simulink model "ControloPosicao2020b"  (R2022b)
settings: Solver=VariableStepAuto  StartTime=0.0  StopTime=10.0  RelTol=1e-3
libraries: fuzblock x12, slpidlib x4, dspswit3 x2
settings Model: Creator=jpmat  LastModifiedBy=jpmat
settings OptimizationCC: ReuseModelBlockBuffer=on

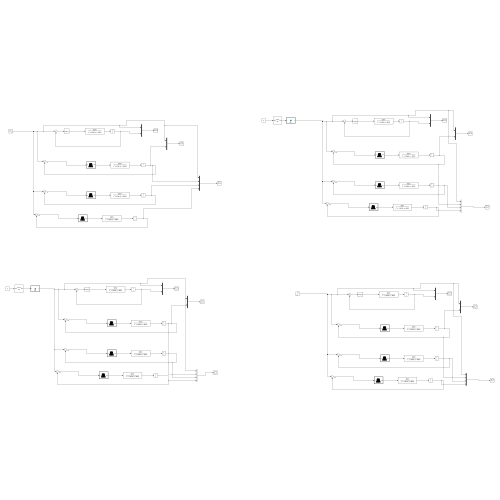
[thumbnail: Simulink's stored preview of the top-level diagram]
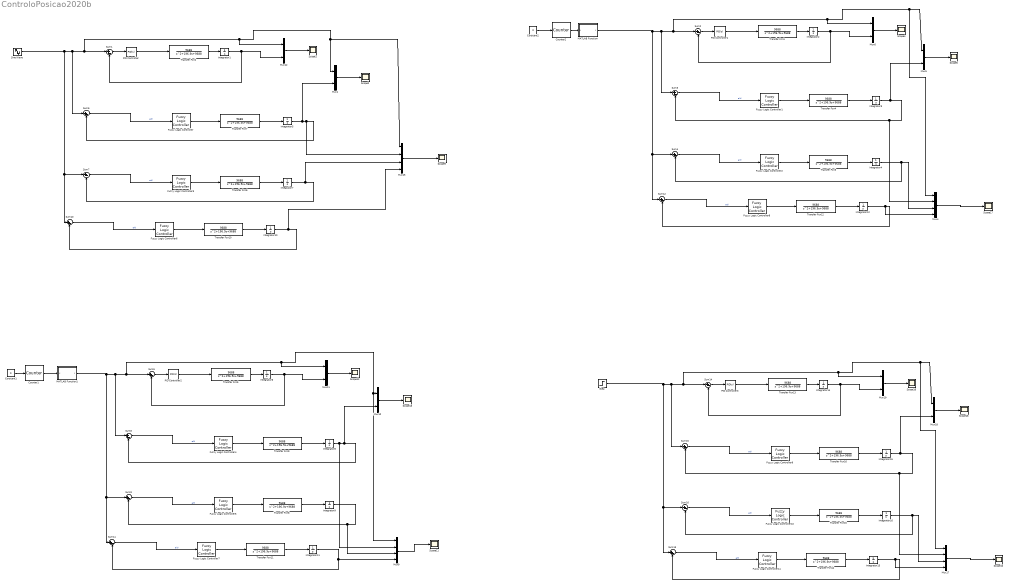
== system ControloPosicao2020b ==
  Constant1 : Constant  Value=0
  Constant2 : Constant  Value=0
  Counter1 : dspswit3/Counter  Direction=Up  CountEvent=Free running  CounterSize=User defined  MaxCount=10000000  InitialCount=0  Output=Count  HitValue=32  ResetInput=on  SamplesPerFrame=1  Ts=0.01  CntDtype=double  HitDtype=Logical
  Counter2 : dspswit3/Counter  Direction=Up  CountEvent=Free running  CounterSize=User defined  MaxCount=10000000  InitialCount=0  Output=Count  HitValue=32  ResetInput=on  SamplesPerFrame=1  Ts=0.01  CntDtype=double  HitDtype=Logical
  Fuzzy Logic Controller{,1,4,9} (4 alike) : fuzblock/Fuzzy Logic  Controller  FIS=posFIS  OutputSampleNumber=101  DataType=double  FuzzifiedInputs=off  RuleFiringStrengths=off  RuleOutputs=off  AggregatedOutputs=off  SimulateUsing=Interpreted execution  OutOfRangeInputValueMessage=warning  NoRuleFiredMessage=warning  EmptyOutputFuzzySetMessage=warning
  Fuzzy Logic Controller{2..3,5,10} (4 alike) : fuzblock/Fuzzy Logic  Controller  FIS=posFIS11  OutputSampleNumber=101  DataType=double  FuzzifiedInputs=off  RuleFiringStrengths=off  RuleOutputs=off  AggregatedOutputs=off  SimulateUsing=Interpreted execution  OutOfRangeInputValueMessage=warning  NoRuleFiredMessage=warning  EmptyOutputFuzzySetMessage=warning
  Fuzzy Logic Controller{6..8,11} (4 alike) : fuzblock/Fuzzy Logic  Controller  FIS=posFIS5  OutputSampleNumber=101  DataType=double  FuzzifiedInputs=off  RuleFiringStrengths=off  RuleOutputs=off  AggregatedOutputs=off  SimulateUsing=Interpreted execution  OutOfRangeInputValueMessage=warning  NoRuleFiredMessage=warning  EmptyOutputFuzzySetMessage=warning
  Integrator{1..16} (16 alike) : Integrator
  MATLAB Function : MATLAB Function  TreatAsAtomicUnit=on
  MATLAB Function1 : MATLAB Function  TreatAsAtomicUnit=on
  Mux{1,5..6,10..12,18..19} (8 alike) : Mux  Inputs=2
  Mux{4,9,15,17} (4 alike) : Mux
  PID Controller{,1..3} (4 alike) : slpidlib/PID Controller  Controller=PID  Form=Parallel  TimeDomain=Continuous-time  UseExternalTs=off  SampleTime=-1  IntegratorMethod=Forward Euler  FilterMethod=Forward Euler  ControllerParametersSource=internal  P=15  I=2  UseKiTs=off  D=0.05  N=100  UseFilter=on  TunerSelectOption=Transfer Function Based (PID Tuner App)  InitialConditionSource=internal  InitialConditionForIntegrator=0  InitialConditionForFilter=0  DifferentiatorICPrevScaledInput=0  ExternalReset=none  TrackingMode=off  Kt=1  LimitOutput=off  SatLimitsSource=internal  UpperSaturationLimit=inf  LowerSaturationLimit=-inf  LinearizeAsGain=on  AntiWindupMode=none  Kb=1  LimitIntegrator=off  UpperIntegratorSaturationLimit=inf  LowerIntegratorSaturationLimit=-inf  POutMin=[]  POutMax=[]  IOutMin=[]  IOutMax=[]  DOutMin=[]  DOutMax=[]  NOutMin=[]  NOutMax=[]  SumOutMin=[]  SumOutMax=[]  SaturationOutMin=[]  SaturationOutMax=[]  PParamMin=[]  PParamMax=[]  IParamMin=[]  IParamMax=[]  DParamMin=[]  DParamMax=[]  NParamMin=[]  NParamMax=[]  KbParamMin=[]  KbParamMax=[]  KtParamMin=[]  KtParamMax=[]  KbOutMin=[]  KbOutMax=[]  KtOutMin=[]  KtOutMax=[]  IntegratorOutMin=[]  IntegratorOutMax=[]  FilterOutMin=[]  FilterOutMax=[]  SumI1OutMin=[]  SumI1OutMax=[]  SumI2OutMin=[]  SumI2OutMax=[]  SumI3OutMin=[]  SumI3OutMax=[]  SumI4OutMin=[]  SumI4OutMax=[]  SumDOutMin=[]  SumDOutMax=[]  DifferentiatorOutMin=[]  DifferentiatorOutMax=[]  FilterDiffOutCoefMin=[]  FilterDiffOutCoefMax=[]  ReciprocalOutMin=[]  ReciprocalOutMax=[]  SumDenOutMin=[]  SumDenOutMax=[]  SumNumOutMin=[]  SumNumOutMax=[]  DivideOutMin=[]  DivideOutMax=[]  UdiffTsProdOutMin=[]  UdiffTsProdOutMax=[]  NTsProdOutMin=[]  NTsProdOutMax=[]  UintegralTsProdOutMin=[]  UintegralTsProdOutMax=[]  UngainTsProdOutMin=[]  UngainTsProdOutMax=[]  IntegratorContinuousStateAttributes=''  IntegratorStateMustResolveToSignalObject=off  IntegratorRTWStateStorageClass=Auto  FilterContinuousStateAttributes=''  FilterStateMustResolveToSignalObject=off  FilterRTWStateStorageClass=Auto  ParallelPVariant=InternalParameters  IdealPVariant=Disabled  IVariant=InternalParameters  DVariant=InternalParameters  IntegratorVariant=Continuous  SatVariant=Disabled  AWVariant=Passthrough  PCopyVariant=Disabled  TRVariant=Disabled  FdbkBlocksVariant=Forward  IdealPFdbkVariant=Disabled  SatFdbkVariant=Disabled  DerivativeFilterVariant=ContFilter  NVariant=InternalParameters  NCopyVariant=Disabled  FilterICVariant=InternalICsFilter  IntegratorICVariant=InternalICs  ExternalResetVariant=Disabled  TRSumVariant=Passthrough  SumFdbkVariant=Disabled  SumVariant=Sum_PID  TsampFilterVariant=InternalTs  TsampNgainVariant=Passthrough  TsampIntegralVariant=Disabled_SignalSpec  ExternalSaturationOutDataTypeStr=Inherit: Same as second input
  Scope{1..2,4..5,9..13,16..18} (12 alike) : Scope
  Sine Wave : Sin  Amplitude=100  Frequency=2*pi()  SampleTime=0
  Step : Step  After=100  SampleTime=0
  Sum{1..16} (16 alike) : Sum  Inputs=|+-
  Transfer Fcn{1..16} (16 alike) : TransferFcn  Numerator=[9688]  Denominator=[1,196.9,9688]
  wires:
  Transfer Fcn7/1 -> Integrator5/1
  Sine Wave/1 -> Sum10/1, Sum7/1, Sum6/1, Mux12/1, Mux1/1, Mux15/1, Sum1/1
  Integrator1/1 -> Sum1/2, Mux12/2
  Sum6/1 -> Fuzzy Logic Controller/1  "e(t)"
  Sum1/1 -> PID Controller/1
  Fuzzy Logic Controller/1 -> Transfer Fcn7/1
  Transfer Fcn2/1 -> Integrator1/1
  PID Controller/1 -> Transfer Fcn2/1
  Integrator5/1 -> Mux1/2, Mux15/2, Sum6/2
  Constant2/1 -> Counter2/1
  Counter2/1 -> MATLAB Function/1(u)
  Integrator7/1 -> Mux15/3, Sum7/2
  Fuzzy Logic Controller3/1 -> Transfer Fcn6/1
  Sum7/1 -> Fuzzy Logic Controller3/1  "e(t)"
  Transfer Fcn6/1 -> Integrator7/1
  Mux1/1 -> Scope2/1
  Constant1/1 -> Counter1/1
  Counter1/1 -> MATLAB Function1/1(u)
  Mux12/1 -> Scope1/1
  Mux6/1 -> Scope4/1
  Mux5/1 -> Scope5/1
  Transfer Fcn3/1 -> Integrator4/1
  Sum4/1 -> Fuzzy Logic Controller2/1  "e(t)"
  Fuzzy Logic Controller2/1 -> Transfer Fcn3/1
  Integrator4/1 -> Mux4/3, Sum4/2
  Integrator3/1 -> Mux4/2, Sum3/2, Mux5/2
  PID Controller1/1 -> Transfer Fcn1/1
  Transfer Fcn1/1 -> Integrator2/1
  Fuzzy Logic Controller1/1 -> Transfer Fcn4/1
  Sum2/1 -> PID Controller1/1
  Sum3/1 -> Fuzzy Logic Controller1/1  "e(t)"
  Integrator2/1 -> Mux6/2, Sum2/2
  MATLAB Function/1(y) -> Sum2/1, Mux4/1, Mux5/1, Mux6/1, Sum3/1, Sum12/1, Sum4/1
  Transfer Fcn4/1 -> Integrator3/1
  Transfer Fcn9/1 -> Integrator8/1
  MATLAB Function1/1(y) -> Sum11/1, Sum9/1, Sum8/1, Mux11/1, Mux9/1, Mux10/1, Sum5/1
  Integrator6/1 -> Sum5/2, Mux11/2
  Sum8/1 -> Fuzzy Logic Controller4/1  "e(t)"
  Sum5/1 -> PID Controller2/1
  Fuzzy Logic Controller4/1 -> Transfer Fcn9/1
  Transfer Fcn5/1 -> Integrator6/1
  PID Controller2/1 -> Transfer Fcn5/1
  Integrator8/1 -> Mux9/2, Mux10/2, Sum8/2
  Integrator9/1 -> Mux9/3, Sum9/2
  Fuzzy Logic Controller5/1 -> Transfer Fcn8/1
  Sum9/1 -> Fuzzy Logic Controller5/1  "e(t)"
  Transfer Fcn8/1 -> Integrator9/1
  Mux10/1 -> Scope13/1
  Mux11/1 -> Scope12/1
  Transfer Fcn10/1 -> Integrator10/1
  Sum10/1 -> Fuzzy Logic Controller6/1  "e(t)"
  Fuzzy Logic Controller6/1 -> Transfer Fcn10/1
  Integrator10/1 -> Mux15/4, Sum10/2
  Mux15/1 -> Scope9/1
  Transfer Fcn11/1 -> Integrator11/1
  Sum11/1 -> Fuzzy Logic Controller7/1  "e(t)"
  Fuzzy Logic Controller7/1 -> Transfer Fcn11/1
  Integrator11/1 -> Mux9/4, Sum11/2
  Mux9/1 -> Scope11/1
  Integrator12/1 -> Mux4/4, Sum12/2
  Fuzzy Logic Controller8/1 -> Transfer Fcn12/1
  Sum12/1 -> Fuzzy Logic Controller8/1  "e(t)"
  Transfer Fcn12/1 -> Integrator12/1
  Mux4/1 -> Scope17/1
  Mux17/1 -> Scope10/1
  Transfer Fcn14/1 -> Integrator13/1
  Sum13/1 -> Fuzzy Logic Controller11/1  "e(t)"
  Fuzzy Logic Controller11/1 -> Transfer Fcn14/1
  Integrator13/1 -> Sum13/2, Mux17/4
  Transfer Fcn16/1 -> Integrator15/1
  Step/1 -> Sum16/1, Sum13/1, Sum15/1, Mux19/1, Mux18/1, Mux17/1, Sum14/1
  Integrator14/1 -> Sum14/2, Mux19/2
  Sum15/1 -> Fuzzy Logic Controller9/1  "e(t)"
  Sum14/1 -> PID Controller3/1
  Fuzzy Logic Controller9/1 -> Transfer Fcn16/1
  Transfer Fcn13/1 -> Integrator14/1
  PID Controller3/1 -> Transfer Fcn13/1
  Integrator15/1 -> Mux18/2, Sum15/2, Mux17/2
  Integrator16/1 -> Sum16/2, Mux17/3
  Fuzzy Logic Controller10/1 -> Transfer Fcn15/1
  Sum16/1 -> Fuzzy Logic Controller10/1  "e(t)"
  Transfer Fcn15/1 -> Integrator16/1
  Mux18/1 -> Scope18/1
  Mux19/1 -> Scope16/1

== matlab function ControloPosicao2020b/MATLAB Function ==
  data: u input; y output
function y = fcn(u)
u=u/100;

if u>=0 && u<1
    y=50*u;
elseif u>=1 && u<1.4918
    y=50;
elseif u>=1.4918 && u<2.539
    y=50*sin(3*u+1.8078)+50;
elseif u>=2.539 && u<3.04
    y=100*(u-2.04);
elseif u>=3.04 && u<4
    y=100;
elseif u>=4 && u<5
    y=-100*(u-5);
elseif u>=5 && u<(5*pi/3)
    y=0;
elseif u>=(5*pi/3) && u<10
    y=50*(sin(3*u)*cos(2*u));
else
    y=0;

end

== matlab function ControloPosicao2020b/MATLAB Function1 ==
  data: u input; y output
function y = fcn(u)
u=u/100;

if u>=0 && u<=0.5
    y=0;

elseif u>0.5 && u<=0.833
    y=300*u-150;

elseif u>0.833 && u<=1.167
    y=-300*u+350;

elseif u>1.167 && u<=1.5
    y=300*u-350;

elseif u>1.5 && u<=1.833
    y=-300*u+550;

else
    y=0;
end
       
    
end
